simulink model "M2"  (R2012b)
settings: Solver=ode45  StartTime=0.0  StopTime=5  RelTol=1e-3
libraries: simulink x1
settings Model: Creator=user  LastModifiedBy=user
settings DebuggingCC: SolverPrmCheckMsg=none

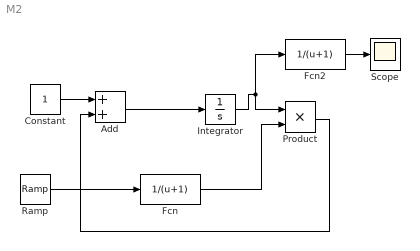
== system M2 ==
  Add : Sum
  Constant : Constant
  Fcn : Fcn  Expr=1/(u+1)
  Fcn2 : Fcn  Expr=1/(u+1)
  Integrator : Integrator
  Product : Product  RndMeth=Zero
  Ramp : simulink/Sources/Ramp  slope=1  start=0  X0=0
  Scope : Scope
  wires:
  Fcn/1 -> Product/2
  Integrator/1 -> Fcn2/1, Product/1
  Product/1 -> Add/2
  Add/1 -> Integrator/1
  Ramp/1 -> Fcn/1
  Fcn2/1 -> Scope/1
  Constant/1 -> Add/1
